simulink model "Lead_Lag_translatorisk_samla"  (R2023b)
settings: Solver=VariableStepAuto  StartTime=0.0  StopTime=1  RelTol=1e-8
values from neighbouring files (symbols this model uses):
  D_hiv_fart = [M(3),rho_vann*Cd*A_z*Z_2]    [Lead_Lag.m]
settings Model: Creator=Anne Brit  LastModifiedBy=anneb
settings DataIOCC: InitialState=0.5

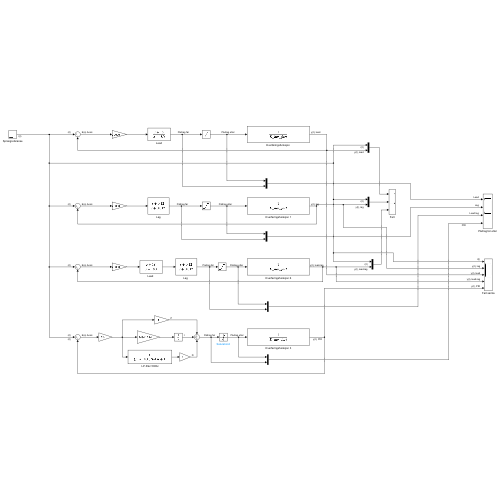
[thumbnail: Simulink's stored preview of the top-level diagram]
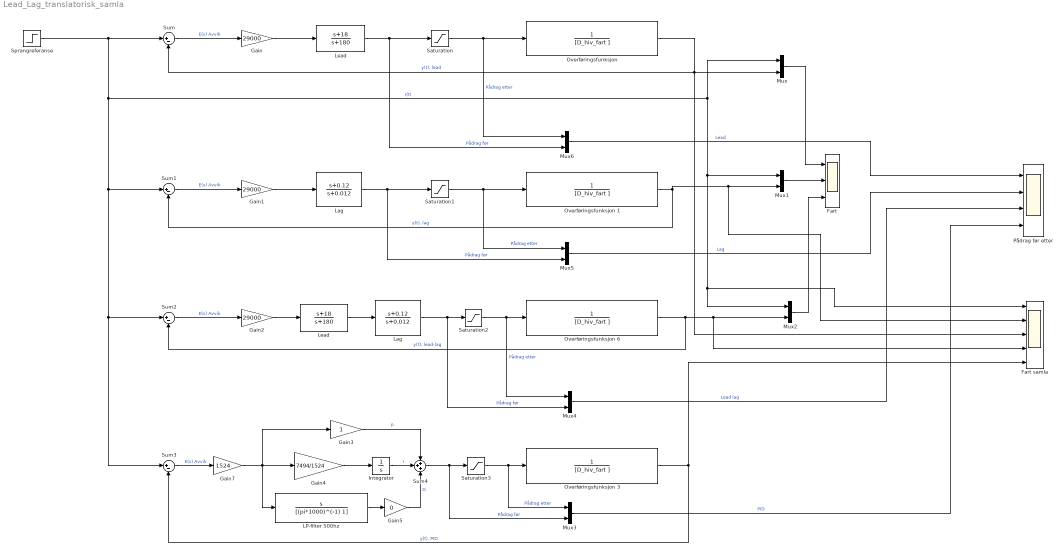
== system Lead_Lag_translatorisk_samla ==
  " LP-filter 500hz" : TransferFcn  Numerator=[1 0]  Denominator=[(pi*1000)^(-1) 1]
  Fart : Scope  NumInputPorts=3
  Fart samla : Scope  NumInputPorts=5
  Gain : Gain  Gain=29000
  Gain1 : Gain  Gain=29000
  Gain2 : Gain  Gain=29000
  Gain3 : Gain
  Gain4 : Gain  Gain=7494/1524
  Gain5 : Gain  Gain=0
  Gain7 : Gain  Gain=1524
  Integrator : Integrator
  Lag : TransferFcn  Numerator=[1 0.12]  Denominator=[1 0.012 ]
  "Lag  " : TransferFcn  Numerator=[1 0.12]  Denominator=[1 0.012 ]
  Lead : TransferFcn  Numerator=[1 18]  Denominator=[1 180 ]
  "Lead  " : TransferFcn  Numerator=[1 18]  Denominator=[1 180 ]
  Mux{,1..6} (7 alike) : Mux  Inputs=2
  Overføringsfunksjon {,1,3,6} (4 alike) : TransferFcn  Denominator=[D_hiv_fart ]
  Pådrag før etter : Scope  NumInputPorts=4
  Saturation{,1..3} (4 alike) : Saturate  UpperLimit=115  LowerLimit=-145
  Sprangreferanse : Step  Time=0.05  After=0.0325  SampleTime=0
  Sum{,1..3} (4 alike) : Sum  Inputs=|+-
  Sum4 : Sum  Inputs=+++
  wires:
  "Overføringsfunksjon "/1 -> Sum/2, Fart samla/3, Mux/2  "y(t), lead"
  Sum/1 -> Gain/1  "E(s) Avvik"
  Saturation/1 -> "Overføringsfunksjon "/1, Mux6/1  "Pådrag etter"
  Lead/1 -> Saturation/1, Mux6/2  "Pådrag før"
  Gain/1 -> Lead/1
  Sum1/1 -> Gain1/1  "E(s) Avvik"
  Overføringsfunksjon 1/1 -> Mux1/2, Fart samla/2, Sum1/2  "y(t), lag"
  Gain1/1 -> Lag/1
  Sum2/1 -> Gain2/1  "E(s) Avvik"
  Overføringsfunksjon 6/1 -> Fart samla/4, Mux2/2, Sum2/2  "y(t), lead-lag"
  "Lead  "/1 -> "Lag  "/1
  Gain2/1 -> "Lead  "/1
  Mux/1 -> Fart/1
  Mux1/1 -> Fart/2
  Mux2/1 -> Fart/3
  Saturation3/1 -> Mux3/1, Overføringsfunksjon 3/1  "Pådrag etter"
  Gain4/1 -> Integrator/1
  " LP-filter 500hz"/1 -> Gain5/1
  Sum4/1 -> Mux3/2, Saturation3/1  "Pådrag før"
  Sprangreferanse/1 -> Mux1/1, Mux2/1, Fart samla/1, Mux/1, Sum3/1, Sum2/1, Sum1/1, Sum/1  "r(t)"
  Gain5/1 -> Sum4/3  "D"
  Gain3/1 -> Sum4/1  "P"
  Sum3/1 -> Gain7/1  "E(s) Avvik"
  Integrator/1 -> Sum4/2  "I"
  Overføringsfunksjon 3/1 -> Fart samla/5, Sum3/2  "y(t), PID"
  Gain7/1 -> Gain3/1, Gain4/1, " LP-filter 500hz"/1
  Saturation2/1 -> Mux4/1, Overføringsfunksjon 6/1  "Pådrag etter"
  "Lag  "/1 -> Mux4/2, Saturation2/1  "Pådrag før"
  Saturation1/1 -> Mux5/1, Overføringsfunksjon 1/1  "Pådrag etter"
  Lag/1 -> Mux5/2, Saturation1/1  "Pådrag før"
  Mux6/1 -> Pådrag før etter/1  "Lead"
  Mux5/1 -> Pådrag før etter/2  "Lag"
  Mux4/1 -> Pådrag før etter/3  "Lead lag"
  Mux3/1 -> Pådrag før etter/4  "PID"
